simulink subsystem "MotorGenerator1Basic_refsub"  (R2022a)
settings: Solver=VariableStepAuto  StartTime=0.0  StopTime=10.0  RelTol=1e-3
undefined symbols (not defined in the file or in its folder): Minus, motorGenerator1, Plus
libraries: fl_lib x8, nesl_utility x6, sdl_lib x1
settings Model: Creator=isaacito  LastModifiedBy=isaacito
settings SolverCC: AlgebraicLoopSolver=TrustRegion
settings DebuggingCC: UnconnectedInputMsg=warning  UnconnectedOutputMsg=warning  UnconnectedLineMsg=warning  SFMachineParentedDataDiag=warning
settings RTWCC: DLArmComputeVersion=19.05

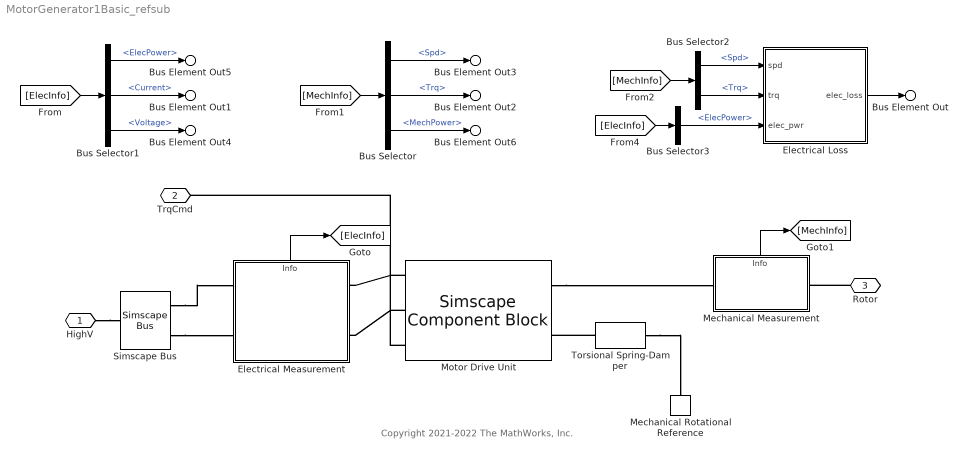
== system MotorGenerator1Basic_refsub ==
  note: Copyright 2021-2022 The MathWorks, Inc.
  Bus Selector : BusSelector  OutputSignals=Spd,Trq,MechPower
  Bus Selector1 : BusSelector  OutputSignals=ElecPower,Current,Voltage
  Bus Selector2 : BusSelector  OutputSignals=Spd,Trq
  Bus Selector3 : BusSelector  OutputSignals=ElecPower
  Electrical Loss : Subsystem
  Electrical Measurement : Subsystem
      settings: PortSchema="{\"entries\":[{\"content\":{\"sides\":[{\"content\":{\"connectorIds\":[\"LConn1\",\"LConn2\"]},\"type\":\"ConnectorPlacement.EquallySpacedRectSide\",\"uuid\":\"9ab4de96-6b59-403f-a104-f6598cec0f44\"},{\"content\":{\"connectorIds\":[\"RConn1\",\"RConn2\"],\"side\":\"RIGHT\"},\"type\":\"ConnectorPlacement.EquallySpacedRectSide\",\"uuid\":\"bacf50cc-d132-4607-ab3e-182152f38282\"},{\"content\":{\"connectorIds\":[\"Out1\"],\"side\":\"TOP\"},\"type\":\"ConnectorPlacement.EquallySpacedRectSide\",\"uuid\":\"783c446a-4d08-439b-a899-02a050ea426b\"},{\"content\":{\"connectorIds\":[],\"side\":\"HIDDEN\"},\"type\":\"ConnectorPlacement.EquallySpacedRectSide\",\"uuid\":\"5928f211-55c3-4dc9-a146-49bbdb386f2a\"}]},\"type\":\"ConnectorPlacement.EquallySpacedConnector\",\"uuid\":\"439f0c16-fbf3-46c0-98fd-18b00cf76358\"}],\"packageUris\":[\"http://schema.mathworks.com/mf0/Connector/R2020b\"],\"version\":\"1.0\"}"
  Mechanical Rotational Reference : fl_lib/Mechanical/Rotational Elements/Mechanical Rotational Reference
      settings: SourceProductBaseCode=PW,SS,VE
  Mechanical Measurement : Subsystem
      settings: PortSchema="{\"entries\":[{\"content\":{\"sides\":[{\"content\":{\"connectorIds\":[\"LConn1\"]},\"type\":\"ConnectorPlacement.EquallySpacedRectSide\",\"uuid\":\"5fa31342-f07e-4673-a9a7-985a7d429b77\"},{\"content\":{\"connectorIds\":[\"RConn1\"],\"side\":\"RIGHT\"},\"type\":\"ConnectorPlacement.EquallySpacedRectSide\",\"uuid\":\"9acd2d80-16ac-46ed-87fd-cbe927805b31\"},{\"content\":{\"connectorIds\":[\"Out1\"],\"side\":\"TOP\"},\"type\":\"ConnectorPlacement.EquallySpacedRectSide\",\"uuid\":\"4cbbe886-3c02-40e0-8c42-e8f0172dc845\"},{\"content\":{\"connectorIds\":[],\"side\":\"HIDDEN\"},\"type\":\"ConnectorPlacement.EquallySpacedRectSide\",\"uuid\":\"587bbe77-2244-497b-b5ee-9581dc02e6d6\"}]},\"type\":\"ConnectorPlacement.EquallySpacedConnector\",\"uuid\":\"7667f692-53dd-486a-a403-194e7923bdd7\"}],\"packageUris\":[\"http://schema.mathworks.com/mf0/Connector/R2020b\"],\"version\":\"1.0\"}"
  Motor Drive Unit : SimscapeComponentBlock  SourceFile=MotorDriveUnitBasic  ComponentPath=MotorDriveUnitBasic  ComponentVariants="[\"MotorDriveUnitBasic\"]"  ComponentVariantNames="[\"MotorDriveUnitBasic\"]"  ClassName=MotorDriveUnitBasic  SchemaVersion=1  trq_max=motorGenerator1.trqMax_Nm N*m  spd_max=motorGenerator1.spdMax_rpm rpm  power_max=motorGenerator1.powerMax_kW kW  response_time_const=motorGenerator1.responseTime_s s  action_spd=simscape.enum.assert.action.warn  efficiency_pct=motorGenerator1.efficiency_pct  spd_eff=motorGenerator1.spd_eff_rpm rpm  trq_eff=motorGenerator1.trq_eff_Nm N*m  iron_to_nominal_ratio=motorGenerator1.iron_loss_to_nominal_ratio  elec_loss_const=motorGenerator1.elecLossConst_W W  J_rotor=motorGenerator1.rotorInertia_kg_m2 kg*m^2  k_damp=motorGenerator1.kDamp_Nm_per_radPerS N*m/(rad/s)  initial_spd=initial.motorGenerator1_speed_rpm rpm
      settings: CopyFcn=simscape.engine.sli.internal.componentblockcallback(gcbh,'COPY')  PreCopyFcn=simscape.engine.sli.internal.componentblockcallback(gcbh,'PRECOPY')  PreDeleteFcn=simscape.engine.sli.internal.componentblockcallback(gcbh,'PREDELETE')  InternalSimscapePortConfiguration="{\"Bottom\":[],\"Left\":[{\"id\":\"Vp\",\"label\":\"Vplus\",\"type\":\"foundation.electrical.electrical\"},{\"id\":\"Vm\",\"label\":\"Vminus\",\"type\":\"foundation.electrical.electrical\"}],\"Right\":[{\"id\":\"R\",\"label\":\"R\",\"type\":\"foundation.mechanical.rotational.rotational\"},{\"id\":\"C\",\"label\":\"C\",\"type\":\"foundation.mechanical.rotational.rotational\"}],\"Top\":[{\"id\":\"trq_in\",\"label\":\"TrqCmd\",\"type\":\"input\"}]}"
      mask Type: Simple Motor Drive Unit
  Simscape Bus : SimscapeBus  HierarchyStrings=Plus;Minus
  Torsional Spring-Damper : sdl_lib/Couplings & Drives/Torsional Spring-Damper  k=motorGenerator1.dampSpringStiffness_Nm_per_rad N*m/rad  mu_visc=motorGenerator1.dampSpringFriction_Nm_per_rpm m*N/rpm  trq_coulomb=0 N*m  static_kinetic_ratio=1.1  w_tol=smoothing.mg1_dampSpringVelTol_rpm rpm  model_hardstop=0  upper_bound=10 deg  lower_bound=-10 deg  k_endstop=1e6 N*m/rad  D_endstop=10 N*m/(rad/s)  hardstop_model=1  transition=0.001 rad  x0=0 deg
      settings: SourceProductBaseCode=LD  InternalSimscapePortConfiguration="{\"Bottom\":[],\"Left\":[{\"id\":\"R\",\"label\":\"R\",\"type\":\"foundation.mechanical.rotational.rotational\"}],\"Right\":[{\"id\":\"C\",\"label\":\"C\",\"type\":\"foundation.mechanical.rotational.rotational\"}],\"Top\":[]}"
  HighV : PMIOPort  Side=Left
  TrqCmd : PMIOPort  Port=2  Side=Left
  Rotor : PMIOPort  Port=3  Side=Right
  Bus Element Out : Outport  PortName=Info  Element=ElecLoss
      settings: AttributesFormatString=%<Unit>
  Bus Element Out1 : Outport  PortName=Info  Element=Current
      settings: AttributesFormatString=%<Unit>
  Bus Element Out2 : Outport  PortName=Info  Element=Trq
      settings: AttributesFormatString=%<Unit>
  Bus Element Out3 : Outport  PortName=Info  Element=Spd
      settings: AttributesFormatString=%<Unit>
  Bus Element Out4 : Outport  PortName=Info  Element=Voltage
      settings: AttributesFormatString=%<Unit>
  Bus Element Out5 : Outport  PortName=Info  Element=ElecPower
      settings: AttributesFormatString=%<Unit>
  Bus Element Out6 : Outport  PortName=Info  Element=MechPower
      settings: AttributesFormatString=%<Unit>
  wires:
  [MechInfo] -> Bus Selector/1
  [ElecInfo] -> Bus Selector3/1
  Electrical Measurement/1(Info) -> [ElecInfo]
  Bus Selector1/1 -> Bus Element Out5/1  "<ElecPower>"
  Bus Selector/1 -> Bus Element Out3/1  "<Spd>"
  [ElecInfo] -> Bus Selector1/1
  Bus Selector3/1 -> Electrical Loss/3(elec_pwr)  "<ElecPower>"
  Bus Selector2/1 -> Electrical Loss/1(spd)  "<Spd>"
  Bus Selector/3 -> Bus Element Out6/1  "<MechPower>"
  Bus Selector2/2 -> Electrical Loss/2(trq)  "<Trq>"
  Electrical Loss/1(elec_loss) -> Bus Element Out/1
  [MechInfo] -> Bus Selector2/1
  Bus Selector/2 -> Bus Element Out2/1  "<Trq>"
  Bus Selector1/2 -> Bus Element Out1/1  "<Current>"
  Mechanical Measurement/1(Info) -> [MechInfo]
  Bus Selector1/3 -> Bus Element Out4/1  "<Voltage>"
  connections:
  Motor Drive Unit/LConn2 -- Electrical Measurement/RConn2
  Motor Drive Unit/RConn1 -- Mechanical Measurement/LConn1
  Simscape Bus/LConn1 -- Electrical Measurement/LConn1
  Rotor/RConn1 -- Mechanical Measurement/RConn1
  Motor Drive Unit/LConn1 -- Electrical Measurement/RConn1
  HighV/RConn1 -- Simscape Bus/RConn1
  Simscape Bus/LConn2 -- Electrical Measurement/LConn2
  Motor Drive Unit/LConn3 -- TrqCmd/RConn1
  Torsional Spring-Damper/LConn1 -- Motor Drive Unit/RConn2
  Torsional Spring-Damper/RConn1 -- Mechanical Rotational Reference/LConn1

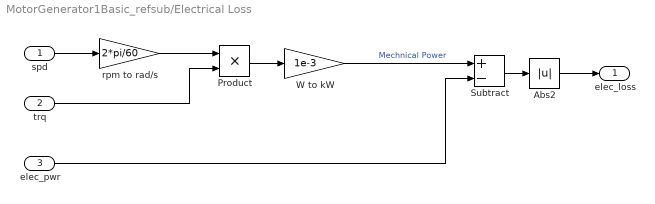
== system MotorGenerator1Basic_refsub/Electrical Loss ==
  spd : Inport  Unit=rpm
      settings: AttributesFormatString=%<Unit>
  trq : Inport  Port=2  Unit=N*m
      settings: AttributesFormatString=%<Unit>
  elec_pwr : Inport  Port=3  Unit=kW
      settings: AttributesFormatString=%<Unit>
  Abs2 : Abs  ZeroCross=off  SaturateOnIntegerOverflow=off
  Product : Product
  Subtract : Sum  Inputs=+-
  W to kW : Gain  Gain=1e-3
  rpm to rad/s : Gain  Gain=2*pi/60
  elec_loss : Outport  Unit=kW
      settings: AttributesFormatString=%<Unit>
  wires:
  trq/1 -> Product/2
  spd/1 -> rpm to rad/s/1
  rpm to rad/s/1 -> Product/1
  Product/1 -> W to kW/1
  elec_pwr/1 -> Subtract/2
  Subtract/1 -> Abs2/1
  Abs2/1 -> elec_loss/1
  W to kW/1 -> Subtract/1  "Mechnical Power"

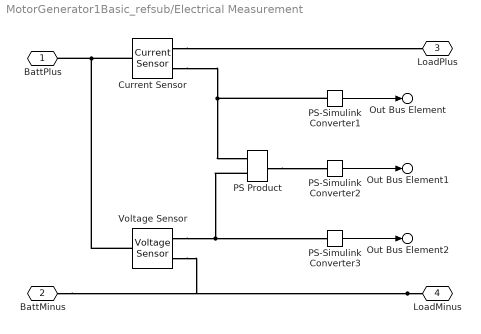
== system MotorGenerator1Basic_refsub/Electrical Measurement ==
  Current Sensor : fl_lib/Electrical/Electrical Sensors/Current Sensor
      settings: SourceProductBaseCode=PW,SS,VE
  PS Product : fl_lib/Physical Signals/Functions/PS Product
      settings: SourceProductBaseCode=PW,SS,VE
  PS-Simulink Converter1 : nesl_utility/PS-Simulink Converter  PhysicalDomain=network_engine_domain  SubClassName=ps_output  LeftPortType=input  RightPortType=output  PseudoPeriodic=off  Frequencies=[]  VectorFormat=1-D array  Unit=A  AffineConversion=off
      settings: SourceProductBaseCode=SS,PW,VE
  PS-Simulink Converter2 : nesl_utility/PS-Simulink Converter  PhysicalDomain=network_engine_domain  SubClassName=ps_output  LeftPortType=input  RightPortType=output  PseudoPeriodic=off  Frequencies=[]  VectorFormat=1-D array  Unit=kW  AffineConversion=off
      settings: SourceProductBaseCode=SS,PW,VE
  PS-Simulink Converter3 : nesl_utility/PS-Simulink Converter  PhysicalDomain=network_engine_domain  SubClassName=ps_output  LeftPortType=input  RightPortType=output  PseudoPeriodic=off  Frequencies=[]  VectorFormat=1-D array  Unit=V  AffineConversion=off
      settings: SourceProductBaseCode=SS,PW,VE
  Voltage Sensor : fl_lib/Electrical/Electrical Sensors/Voltage Sensor
      settings: SourceProductBaseCode=PW,SS,VE
  BattPlus : PMIOPort  Side=Left
  BattMinus : PMIOPort  Port=2  Side=Left
  LoadPlus : PMIOPort  Port=3  Side=Right
  LoadMinus : PMIOPort  Port=4  Side=Right
  Out Bus Element : Outport  PortName=Info  Element=Current
  Out Bus Element1 : Outport  PortName=Info  Element=ElecPower
  Out Bus Element2 : Outport  PortName=Info  Element=Voltage
  wires:
  PS-Simulink Converter3/1 -> Out Bus Element2/1
  PS-Simulink Converter2/1 -> Out Bus Element1/1
  PS-Simulink Converter1/1 -> Out Bus Element/1
  connections:
  PS Product/RConn1 -- PS-Simulink Converter2/LConn1
  PS-Simulink Converter1/LConn1 -- Current Sensor/RConn1 -- PS Product/LConn1
  Current Sensor/RConn2 -- LoadPlus/RConn1
  Voltage Sensor/LConn1 -- Current Sensor/LConn1 -- BattPlus/RConn1
  LoadMinus/RConn1 -- Voltage Sensor/RConn2 -- BattMinus/RConn1
  PS Product/LConn2 -- Voltage Sensor/RConn1 -- PS-Simulink Converter3/LConn1

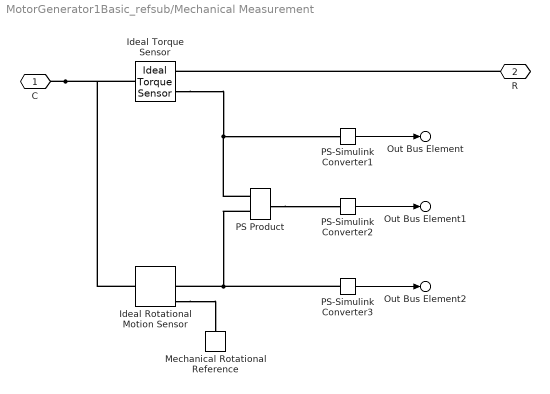
== system MotorGenerator1Basic_refsub/Mechanical Measurement ==
  Ideal Rotational Motion Sensor : fl_lib/Mechanical/Mechanical Sensors/Ideal Rotational Motion Sensor  wrap_angle=simscape.enum.onoff.off  offset=0 rad
      settings: SourceProductBaseCode=PW,SS,VE
  Ideal Torque Sensor : fl_lib/Mechanical/Mechanical Sensors/Ideal Torque Sensor
      settings: SourceProductBaseCode=PW,SS,VE
  Mechanical Rotational Reference : fl_lib/Mechanical/Rotational Elements/Mechanical Rotational Reference
      settings: SourceProductBaseCode=PW,SS,VE
  PS Product : fl_lib/Physical Signals/Functions/PS Product
      settings: SourceProductBaseCode=PW,SS,VE
  PS-Simulink Converter1 : nesl_utility/PS-Simulink Converter  PhysicalDomain=network_engine_domain  SubClassName=ps_output  LeftPortType=input  RightPortType=output  PseudoPeriodic=off  Frequencies=[]  VectorFormat=1-D array  Unit=N*m  AffineConversion=off
      settings: SourceProductBaseCode=SS,PW,VE
  PS-Simulink Converter2 : nesl_utility/PS-Simulink Converter  PhysicalDomain=network_engine_domain  SubClassName=ps_output  LeftPortType=input  RightPortType=output  PseudoPeriodic=off  Frequencies=[]  VectorFormat=1-D array  Unit=kW  AffineConversion=off
      settings: SourceProductBaseCode=SS,PW,VE
  PS-Simulink Converter3 : nesl_utility/PS-Simulink Converter  PhysicalDomain=network_engine_domain  SubClassName=ps_output  LeftPortType=input  RightPortType=output  PseudoPeriodic=off  Frequencies=[]  VectorFormat=1-D array  Unit=rpm  AffineConversion=off
      settings: SourceProductBaseCode=SS,PW,VE
  C : PMIOPort  Side=Left
  R : PMIOPort  Port=2  Side=Right
  Out Bus Element : Outport  PortName=Info  Element=Trq
  Out Bus Element1 : Outport  PortName=Info  Element=MechPower
  Out Bus Element2 : Outport  PortName=Info  Element=Spd
  wires:
  PS-Simulink Converter3/1 -> Out Bus Element2/1
  PS-Simulink Converter2/1 -> Out Bus Element1/1
  PS-Simulink Converter1/1 -> Out Bus Element/1
  connections:
  PS Product/RConn1 -- PS-Simulink Converter2/LConn1
  PS Product/LConn1 -- Ideal Torque Sensor/RConn2 -- PS-Simulink Converter1/LConn1
  R/RConn1 -- Ideal Torque Sensor/RConn1
  C/RConn1 -- Ideal Rotational Motion Sensor/LConn1 -- Ideal Torque Sensor/LConn1
  Ideal Rotational Motion Sensor/RConn1 -- Mechanical Rotational Reference/LConn1
  PS Product/LConn2 -- PS-Simulink Converter3/LConn1 -- Ideal Rotational Motion Sensor/RConn2
